simulink model "ES210A_EcuTMeas"  (R2013b)
settings: Solver=FixedStepDiscrete  SolverMode=SingleTasking  StartTime=0.0  StopTime=1  FixedStep=0.002  RelTol=1e-3
undefined symbols (not defined in the file): ARCHGLBPRM_100MILLISEC_SEC_F32, EcuTFild, EcuTMeasDftT, EcuTMeasFilTau, EcuTMeasNtc0x045FailStep, EcuTMeasNtc0x045PassStep, EcuTMeasRngDiagcMax, EcuTMeasRngDiagcMin, EcuTMeasScag, EcuTMeasScagOffs, NtcSts1, sigbuilder_block
libraries: simulink x2
settings Model: Creator=pz79n7  LastModifiedBy=NZG49T
settings SolverCC: AutoInsertRateTranBlk=on  InsertRTBMode=Always
settings DataIOCC: LimitDataPoints=off  SaveFormat=Structure  ReturnWorkspaceOutputs=on
settings OptimizationCC: BlockReduction=off  InlineParams=on  ZeroExternalMemoryAtStartup=off  ZeroInternalMemoryAtStartup=off  OptimizeModelRefInitCode=on  LifeSpan=1
settings DebuggingCC: SignalInfNanChecking=error  SignalRangeChecking=warning  UnderspecifiedInitializationDetection=Simplified  SolverPrmCheckMsg=error  InheritedTsInSrcMsg=error  DiscreteInheritContinuousMsg=error  SingleTaskRateTransMsg=error  TasksWithSamePriorityMsg=error  SigSpecEnsureSampleTimeMsg=error  CheckMatrixSingularityMsg=error  ParameterUnderflowMsg=error  ParameterPrecisionLossMsg=error  ParameterTunabilityLossMsg=error  FixptConstUnderflowMsg=warning  FixptConstOverflowMsg=warning  VectorMatrixConversionMsg=error  SignalLabelMismatchMsg=error  UnconnectedInputMsg=error  UnconnectedOutputMsg=error  UnconnectedLineMsg=error  SFcnCompatibilityMsg=error  UniqueDataStoreMsg=warning  BusObjectLabelMismatch=error  RootOutportRequireBusObject=error  AssertControl=DisableAll  ModelReferenceIOMsg=error  ModelReferenceVersionMismatchMessage=warning  ModelReferenceIOMismatchMessage=error  ModelReferenceCSMismatchMessage=warning  ModelReferenceDataLoggingMessage=error  StateNameClashWarn=warning  StrictBusMsg=ErrorOnBusTreatedAsVector  NonBusSignalsTreatedAsBus=error  SFUnexpectedBacktrackingDiag=error  SFInvalidInputDataAccessInChartInitDiag=error  SFNoUnconditionalDefaultTransitionDiag=error  SFTransitionOutsideNaturalParentDiag=error  SFUnconditionalTransitionShadowingDiag=error  SFUndirectedBroadcastEventsDiag=error
settings ModelReferenceCC: ModelReferenceNumInstancesAllowed=Single
settings RTWCC: SystemTargetFile=autosar.tlc  GenCodeOnly=on  TemplateMakefile=ert_default_tmf  Description=AUTOSAR  GenerateReport=on  ProcessScript=autosar_make_rtw_hook  LaunchReport=on
settings CodeAppCC: GenerateComments=off  IgnoreCustomStorageClasses=off  CustomSymbolStrType=$N$R$M  CustomSymbolStrBlkIO=$N$M  SimulinkBlockComments=off
settings STFCustomTargetCC: ParMdlRefBuildCompliant=on  CompOptLevelCompliant=on  IncludeMdlTerminateFcn=off  CombineOutputUpdateFcns=on  SuppressErrorStatus=on  ERTFirstTimeCompliant=on  ERTCustomFileBanners=on  SupportNonFinite=off  SupportComplex=off  SupportContinuousTime=off  SupportNonInlinedSFcns=off  MATLABClassNameForMDSCustomization=Simulink.SoftwareTarget.ERTCustomization  AutosarCompliant=on  GRTInterface=off  SystemTargetFile=autosar.tlc
settings ERTTargetCC: CodeReplacementLibrary=ANSI_C  ConcurrentExecutionCompliant=off  IncludeMdlTerminateFcn=off  SuppressErrorStatus=on  SupportNonFinite=off  SupportComplex=off  ModelStepFunctionPrototypeControlCompliant=off  CPPClassGenCompliant=off  AutosarCompliant=on  InlinedParameterPlacement=NonHierarchical  ERTCustomFileTemplate=example_file_process.tlc  EnableUserReplacementTypes=on

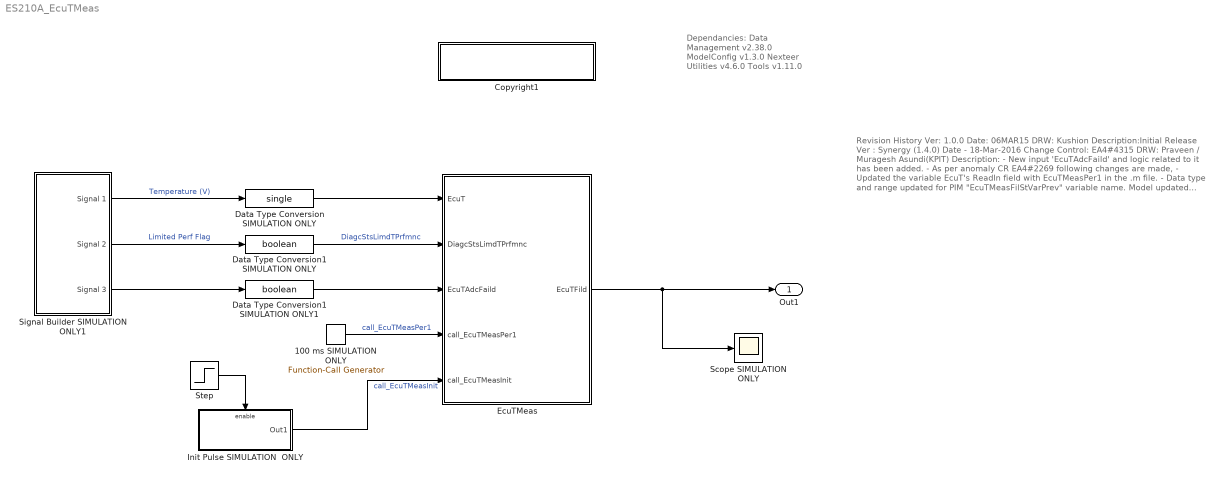
== system ES210A_EcuTMeas ==
  note: Dependancies:
      |    Data Management v2.38.0
      |    ModelConfig v1.3.0
      |    Nexteer Utilities v4.6.0
      |    Tools v1.11.0
  note: Revision History
      |
      | Ver: 1.0.0
      | Date: 06MAR15
      | DRW: Kushion
      | Description:Initial Release
      |
      | Ver : Synergy (1.4.0)
      | Date - 18-Mar-2016
      | Change Control: EA4#4315
      | DRW: Praveen / Muragesh Asundi(KPIT)
      | Description:
      | - New input 'EcuTAdcFaild' and logic related to it has been added.
      | -  As per anomaly CR EA4#2269 following changes are made,
      |   - Updated the variable EcuT's ReadIn field with EcuTMeasPer1 in the .m file.
      |   - Data type and range updated for PIM "EcuTMeasFilStVarPrev" variable name.
      |     Model updated accordingly
      |  - Global constant ARCHGLBPRM_100MILLISEC_SEC_F32 added
      |  - Requirements links updated
      |
      | Ver : 1.4.1
      | Date - 24-Mar-2016
      | Change Control: EA4#4947
      | DRW: Muragesh Asundi(KPIT)
      | New input 'EcuTAdcFaild' added in Data Dict
      |
      | Ver : 1.5.0
      | Date - 28-Apr-2016
      | Change Control: EA4#5549
      | DRW: Samanth Kumaraswamy
      | Changed the incorrect NTC number to 0x45
      | Changed .m file to reflect changes mentioned in the anomaly
      | Added new SetNtcSts Block for DebType for MIL Coverage
  100 ms SIMULATION ONLY : simulink/Ports & Subsystems/Function-Call Generator  sample_time=0.1  numberOfIterations=1
  Copyright1 : Subsystem  Description=|  mask(Copyright Information){none=on}
      | Copyright info block.                                               
      |                                                                     
      | Place copyright information at the top of every subsystem in design.
      mask prompts: none "No parameters"
      mask help: Place copyright information at the top of every subsystem in design.
      mask Display:
      | NxtrConf = 'Nexteer Confidential';
      | 
      | sys = bdroot; %handle for the current model ("system")
      | first = get_param(sys,'Created');
      | if(isempty(first))
      |     first = datestr(now,'yyyy');
      | else
      |     first = first(end-3:end);  %year is last four digits
      | end
      | 
      | last = get_param(sys,'LastModifiedDate');
      | if isempty(last)
      |     last = datestr(now,'yyyy');
      | else
      |     last = last(end-3:end);
      | end
      | 
      | if strcmp(first,last)
      |     fprintf('%s\nCopyright  %s Nexteer',NxtrConf,first);
      | else
      |     fprintf('%s\n%s%s-%s Nexteer',NxtrConf,char(169),first,last);
      | end
  Data Type Conversion SIMULATION ONLY : DataTypeConversion  OutDataTypeStr=single
  Data Type Conversion1 SIMULATION ONLY : DataTypeConversion  OutDataTypeStr=boolean
  Data Type Conversion1 SIMULATION ONLY1 : DataTypeConversion  OutDataTypeStr=boolean
  EcuTMeas : Subsystem
      settings: AttributesFormatString=ES210A
  Init Pulse SIMULATION  ONLY : Subsystem  TreatAsAtomicUnit=on
  Scope SIMULATION ONLY : Scope
      settings: YMin=-50  YMax=150
  Signal Builder SIMULATION ONLY1 : Subsystem  Tag=STV Subsys  LoadFcn=sigbuilder_block('load');  StartFcn=sigbuilder_block('start');  StopFcn=sigbuilder_block('stop');  ClipboardFcn=sigbuilder_block('clipboard');  mask(Sigbuilder block){}
      mask help: Simulink:masks:SigbuilderBlock_MD
      mask init:
      | if ~strcmp(get_param(bdroot(gcbh),'SimulationStatus'),'stopped') tuvar = sigbuilder_block('maskInit'); end
      settings: CopyFcn=sigbuilder_block('copy');  DeleteFcn=sigbuilder_block('delete');  ModelCloseFcn=sigbuilder_block('modelClose');  PreSaveFcn=sigbuilder_block('preSave');  PauseFcn=sigbuilder_block('pause');  ContinueFcn=sigbuilder_block('continue');  NameChangeFcn=sigbuilder_block('namechange');  OpenFcn=sigbuilder_block('open',[33 175.5 591 337.5 ]);  CloseFcn=sigbuilder_block('close');
      mask Display: plot(0, 0, 100, 100,[2, 2, 32, 32, 2], [68, 8, 8, 68, 68],[32, 2], [38, 38], [32, 19, 2],[53, 60, 44], [32, 17, 17, 2],[16, 16, 31, 31]);txt = getActiveGroup(gcbh);text(2, 100, txt,'verticalAlignment', 'top');
  Step : Step  Time=0.002  Before=1  After=0  SampleTime=0
  Out1 : Outport
  wires:
  Signal Builder SIMULATION ONLY1/1(Signal 1) -> Data Type Conversion SIMULATION ONLY/1  "Temperature (V)"
  Signal Builder SIMULATION ONLY1/2(Signal 2) -> Data Type Conversion1 SIMULATION ONLY/1  "Limited Perf Flag"
  100 ms SIMULATION ONLY/1 -> EcuTMeas/4(call_EcuTMeasPer1)  "call_EcuTMeasPer1"
  Step/1 -> Init Pulse SIMULATION  ONLY/Enable
  Init Pulse SIMULATION  ONLY/1(Out1) -> EcuTMeas/5(call_EcuTMeasInit)  "call_EcuTMeasInit"
  Data Type Conversion SIMULATION ONLY/1 -> EcuTMeas/1(EcuT)
  Data Type Conversion1 SIMULATION ONLY/1 -> EcuTMeas/2(DiagcStsLimdTPrfmnc)  "DiagcStsLimdTPrfmnc"
  EcuTMeas/1(EcuTFild) -> Scope SIMULATION ONLY/1, Out1/1
  Signal Builder SIMULATION ONLY1/3(Signal 3) -> Data Type Conversion1 SIMULATION ONLY1/1
  Data Type Conversion1 SIMULATION ONLY1/1 -> EcuTMeas/3(EcuTAdcFaild)

== system ES210A_EcuTMeas/Copyright1 ==

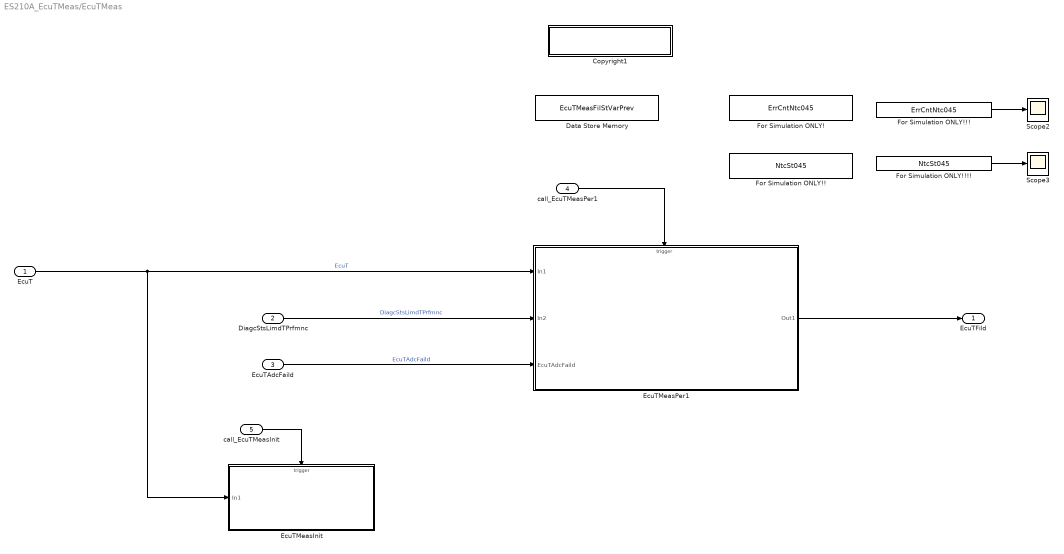
== system ES210A_EcuTMeas/EcuTMeas ==
  EcuT : Inport  RequirementInfo={'linktype_rmi_doors' '000089bf (/E-STEER Core/SubSystem Specifications/Electrical Actuator/Control Module/FDD Module Requirements/EA4/ES210A_EcuTMeas)' '#ES210A_48' 'true' 'REQ: ES210A_48' '' } %GIDa_562c6c3c_e149_4b8a_bc2f_eb7571733cee
  DiagcStsLimdTPrfmnc : Inport  RequirementInfo={'linktype_rmi_doors' '000089bf (/E-STEER Core/SubSystem Specifications/Electrical Actuator/Control Module/FDD Module Requirements/EA4/ES210A_EcuTMeas)' '#ES210A_71' 'true' 'REQ: ES210A_71' '' } %GIDa_c32b2e62_ca29_48d9_a45f_43e18439e176  Port=2
  EcuTAdcFaild : Inport  RequirementInfo={'linktype_rmi_doors' '000089bf (/E-STEER Core/SubSystem Specifications/Electrical Actuator/Control Module/FDD Module Requirements/EA4/ES210A_EcuTMeas)' '#ES210A_82' 'true' 'REQ: ES210A_82' '' } %GIDa_33c9adb4_3b4d_41a0_b691_c5854dca2733  Port=3
  call_EcuTMeasPer1 : Inport  RequirementInfo={'linktype_rmi_doors' '000089bf (/E-STEER Core/SubSystem Specifications/Electrical Actuator/Control Module/FDD Module Requirements/EA4/ES210A_EcuTMeas)' '#ES210A_81' 'true' 'REQ: ES210A_81' '' ; 'linktype_rmi_doors' '000089bf (/E-STEER Core/SubSystem Specifications/Electrical Actuator/Control Module/FDD Module Requirements/EA4/ES210A_EcuTMeas)' '#ES210A_25' 'true' 'REQ: ES210A_25' '' } %GIDa_ca696ddf_736a_4d4a_b70f_f10e14ff3279  Port=4
  call_EcuTMeasInit : Inport  Port=5
  Copyright1 : Subsystem  Description=|  mask(Copyright Information){none=on}
      | Copyright info block.                                               
      |                                                                     
      | Place copyright information at the top of every subsystem in design.
      mask prompts: none "No parameters"
      mask help: Place copyright information at the top of every subsystem in design.
      mask Display:
      | NxtrConf = 'Nexteer Confidential';
      | 
      | sys = bdroot; %handle for the current model ("system")
      | first = get_param(sys,'Created');
      | if(isempty(first))
      |     first = datestr(now,'yyyy');
      | else
      |     first = first(end-3:end);  %year is last four digits
      | end
      | 
      | last = get_param(sys,'LastModifiedDate');
      | if isempty(last)
      |     last = datestr(now,'yyyy');
      | else
      |     last = last(end-3:end);
      | end
      | 
      | if strcmp(first,last)
      |     fprintf('%s\nCopyright  %s Nexteer',NxtrConf,first);
      | else
      |     fprintf('%s\n%s%s-%s Nexteer',NxtrConf,char(169),first,last);
      | end
  Data Store Memory : DataStoreMemory  DataStoreName=EcuTMeasFilStVarPrev  InitialValue=struct('FilSt',single(0),'FilGain',single(0))  OutDataTypeStr=Bus: FilLpRec1  StateMustResolveToSignalObject=on
  EcuTMeasInit : Subsystem  RequirementInfo={'linktype_rmi_doors' '000089bf (/E-STEER Core/SubSystem Specifications/Electrical Actuator/Control Module/FDD Module Requirements/EA4/ES210A_EcuTMeas)' '#ES210A_80' 'true' 'REQ: ES210A_80' '' } %GIDa_ede09633_558d_45b8_b146_d426592bfdd4  TreatAsAtomicUnit=on
  EcuTMeasPer1 : Subsystem  TreatAsAtomicUnit=on
  For Simulation ONLY! : DataStoreMemory  DataStoreName=ErrCntNtc045
  For Simulation ONLY!! : DataStoreMemory  DataStoreName=NtcSt045  OutDataTypeStr=uint8
  For Simulation ONLY!!! : DataStoreRead  DataStoreName=ErrCntNtc045  SampleTime=0.1
  For Simulation ONLY!!!! : DataStoreRead  DataStoreName=NtcSt045  SampleTime=0.1
  Scope2 : Scope
      settings: YMin=-35000  YMax=35000  SaveName=ScopeData2  MaxDataPoints=20000
  Scope3 : Scope
      settings: YMin=-35000  YMax=5000  SaveName=ScopeData4  MaxDataPoints=20000
  EcuTFild : Outport  RequirementInfo={'linktype_rmi_doors' '000089bf (/E-STEER Core/SubSystem Specifications/Electrical Actuator/Control Module/FDD Module Requirements/EA4/ES210A_EcuTMeas)' '#ES210A_51' 'true' 'REQ: ES210A_51' '' } %GIDa_e5beccf4_d72f_4678_b409_538621bbf562
  wires:
  EcuT/1 -> EcuTMeasInit/1(In1), EcuTMeasPer1/1(In1)  "EcuT"
  DiagcStsLimdTPrfmnc/1 -> EcuTMeasPer1/2(In2)  "DiagcStsLimdTPrfmnc"
  EcuTMeasPer1/1(Out1) -> EcuTFild/1
  call_EcuTMeasPer1/1 -> EcuTMeasPer1/Trigger
  call_EcuTMeasInit/1 -> EcuTMeasInit/Trigger
  For Simulation ONLY!!!/1 -> Scope2/1
  For Simulation ONLY!!!!/1 -> Scope3/1
  EcuTAdcFaild/1 -> EcuTMeasPer1/3(EcuTAdcFaild)  "EcuTAdcFaild"

== system ES210A_EcuTMeas/Init Pulse SIMULATION  ONLY ==
  Enable : EnablePort
  "0.002 " : simulink/Ports & Subsystems/Function-Call Generator  sample_time=0.002  numberOfIterations=1
  Copyright1 : Subsystem  Description=|  mask(Copyright Information){none=on}
      | Copyright info block.                                               
      |                                                                     
      | Place copyright information at the top of every subsystem in design.
      mask prompts: none "No parameters"
      mask help: Place copyright information at the top of every subsystem in design.
      mask Display:
      | NxtrConf = 'Nexteer Confidential';
      | 
      | sys = bdroot; %handle for the current model ("system")
      | first = get_param(sys,'Created');
      | if(isempty(first))
      |     first = datestr(now,'yyyy');
      | else
      |     first = first(end-3:end);  %year is last four digits
      | end
      | 
      | last = get_param(sys,'LastModifiedDate');
      | if isempty(last)
      |     last = datestr(now,'yyyy');
      | else
      |     last = last(end-3:end);
      | end
      | 
      | if strcmp(first,last)
      |     fprintf('%s\nCopyright  %s Nexteer',NxtrConf,first);
      | else
      |     fprintf('%s\n%s%s-%s Nexteer',NxtrConf,char(169),first,last);
      | end
  Out1 : Outport
  wires:
  "0.002 "/1 -> Out1/1

== system ES210A_EcuTMeas/Signal Builder SIMULATION ONLY1 ==
  Demux : Demux  Tag=STV Demux  Outputs=3
  FromWs : FromWorkspace  Tag=STV FromWs  VariableName=tuvar  SampleTime=0
      SigBuilderData=|
      | common.afterFinalStr = 'Extrapolate'
      | common.sampleTime = 0
      | dataSet.timeRange = [0 20]
      | dataSet.name = 'Group 1'
      | sbobj.Groups.Name = 'Group 1'
      | sbobj.Groups.Signals(1).Name = 'Signal 1'
      | sbobj.Groups.Signals(1).XData = [0 0.44 0.44 4.05 6 10 20]
      | sbobj.Groups.Signals(1).YData = [0.1 0.1 2 1.98 0 -0.02 0.98]
      | sbobj.Groups.Signals(2).Name = 'Signal 2'
      | sbobj.Groups.Signals(2).XData = [0 12 12 16 16 20]
      | sbobj.Groups.Signals(2).YData = [0 0 1 1 0 0]
      | sbobj.Groups.Signals(3).Name = 'Signal 3'
      | sbobj.Groups.Signals(3).XData = [0 10 10 20]
      | sbobj.Groups.Signals(3).YData = [0 0 1 1]
      | sbobj.Groups.TimeRange = [0 20]
  Signal 1 : Outport  Tag=STV Outport
  Signal 2 : Outport  Tag=STV Outport  Port=2
  Signal 3 : Outport  Tag=STV Outport  Port=3
  wires:
  Demux/1 -> Signal 1/1
  FromWs/1 -> Demux/1
  Demux/2 -> Signal 2/1
  Demux/3 -> Signal 3/1

== system ES210A_EcuTMeas/EcuTMeas/Copyright1 ==

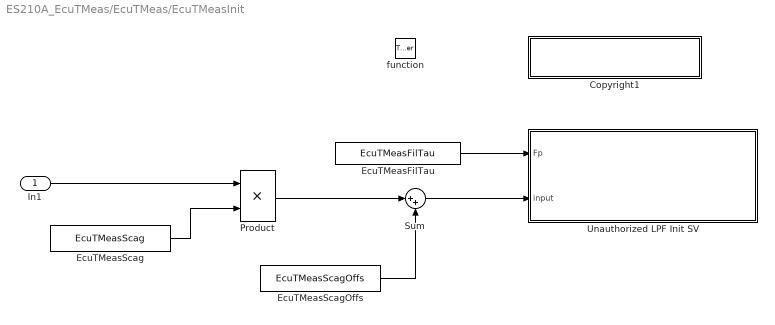
== system ES210A_EcuTMeas/EcuTMeas/EcuTMeasInit ==
  In1 : Inport
  function : TriggerPort  TriggerType=function-call
  Copyright1 : Subsystem  Description=|  mask(Copyright Information){none=on}
      | Copyright info block.                                               
      |                                                                     
      | Place copyright information at the top of every subsystem in design.
      mask prompts: none "No parameters"
      mask help: Place copyright information at the top of every subsystem in design.
      mask Display:
      | NxtrConf = 'Nexteer Confidential';
      | 
      | sys = bdroot; %handle for the current model ("system")
      | first = get_param(sys,'Created');
      | if(isempty(first))
      |     first = datestr(now,'yyyy');
      | else
      |     first = first(end-3:end);  %year is last four digits
      | end
      | 
      | last = get_param(sys,'LastModifiedDate');
      | if isempty(last)
      |     last = datestr(now,'yyyy');
      | else
      |     last = last(end-3:end);
      | end
      | 
      | if strcmp(first,last)
      |     fprintf('%s\nCopyright  %s Nexteer',NxtrConf,first);
      | else
      |     fprintf('%s\n%s%s-%s Nexteer',NxtrConf,char(169),first,last);
      | end
  EcuTMeasFilTau : Constant  RequirementInfo={'linktype_rmi_doors' '000089bf (/E-STEER Core/SubSystem Specifications/Electrical Actuator/Control Module/FDD Module Requirements/EA4/ES210A_EcuTMeas)' '#ES210A_67' 'true' 'REQ: ES210A_67' '' } %GIDa_f1dce8fb_aef4_4cc7_a37f_61aa5bf3e739  Value=EcuTMeasFilTau
  EcuTMeasScag : Constant  RequirementInfo={} %GIDa_ff96598e_3599_4953_8511_9f6c43a5e0a1  Value=EcuTMeasScag
  EcuTMeasScagOffs : Constant  RequirementInfo={} %GIDa_8b7473a9_4ab2_46d8_9d94_f7d56c34d4f4  Value=EcuTMeasScagOffs
  Product : Product  RequirementInfo={} %GIDa_a162ff9c_cdae_4af1_a9a0_ea0d92bfda14
  Sum : Sum  RequirementInfo={} %GIDa_ba1681a0_b4a7_47a3_b5b1_4ffa2c281a80  Inputs=|++
  Unauthorized LPF Init SV : Subsystem
  wires:
  EcuTMeasFilTau/1 -> Unauthorized LPF Init SV/1(Fp)
  In1/1 -> Product/1
  EcuTMeasScag/1 -> Product/2
  Product/1 -> Sum/1
  EcuTMeasScagOffs/1 -> Sum/2
  Sum/1 -> Unauthorized LPF Init SV/2(input)

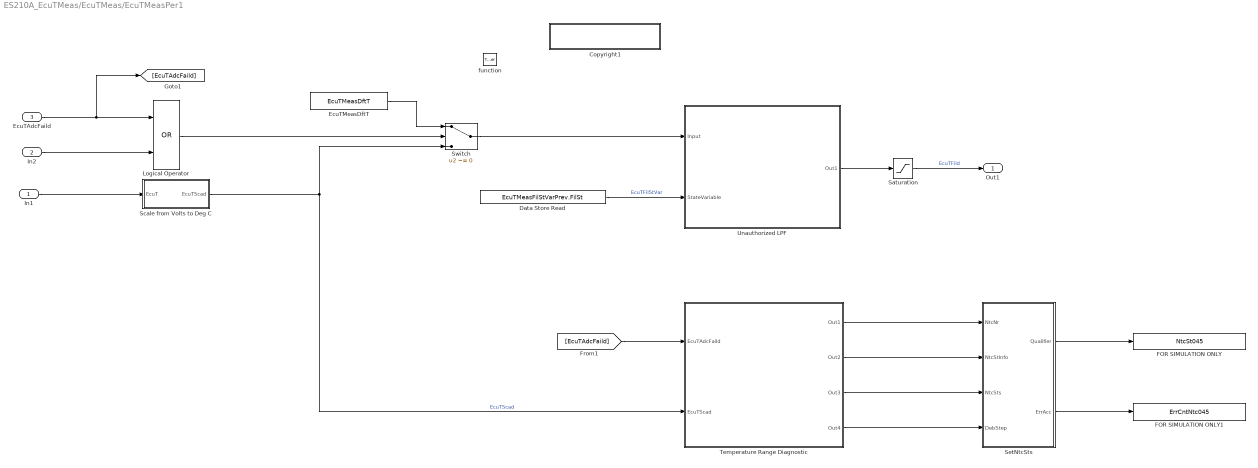
== system ES210A_EcuTMeas/EcuTMeas/EcuTMeasPer1 ==
  In1 : Inport
  In2 : Inport  Port=2
  EcuTAdcFaild : Inport  Port=3
  function : TriggerPort  TriggerType=function-call
  Copyright1 : Subsystem  Description=|  mask(Copyright Information){none=on}
      | Copyright info block.                                               
      |                                                                     
      | Place copyright information at the top of every subsystem in design.
      mask prompts: none "No parameters"
      mask help: Place copyright information at the top of every subsystem in design.
      mask Display:
      | NxtrConf = 'Nexteer Confidential';
      | 
      | sys = bdroot; %handle for the current model ("system")
      | first = get_param(sys,'Created');
      | if(isempty(first))
      |     first = datestr(now,'yyyy');
      | else
      |     first = first(end-3:end);  %year is last four digits
      | end
      | 
      | last = get_param(sys,'LastModifiedDate');
      | if isempty(last)
      |     last = datestr(now,'yyyy');
      | else
      |     last = last(end-3:end);
      | end
      | 
      | if strcmp(first,last)
      |     fprintf('%s\nCopyright  %s Nexteer',NxtrConf,first);
      | else
      |     fprintf('%s\n%s%s-%s Nexteer',NxtrConf,char(169),first,last);
      | end
  Data Store Read : DataStoreRead  DataStoreName=EcuTMeasFilStVarPrev  DataStoreElements=EcuTMeasFilStVarPrev.FilSt
  EcuTMeasDftT : Constant  RequirementInfo={'linktype_rmi_doors' '000089bf (/E-STEER Core/SubSystem Specifications/Electrical Actuator/Control Module/FDD Module Requirements/EA4/ES210A_EcuTMeas)' '#ES210A_84' 'true' 'REQ: ES210A_84' '' } %GIDa_b1347350_8d2d_43af_8bf2_ecc8e1b64997  Value=EcuTMeasDftT
  FOR SIMULATION ONLY : DataStoreWrite  DataStoreName=NtcSt045
  FOR SIMULATION ONLY1 : DataStoreWrite  DataStoreName=ErrCntNtc045
  Logical Operator : Logic  RequirementInfo={'linktype_rmi_doors' '000089bf (/E-STEER Core/SubSystem Specifications/Electrical Actuator/Control Module/FDD Module Requirements/EA4/ES210A_EcuTMeas)' '#ES210A_84' 'true' 'REQ: ES210A_84' '' } %GIDa_55355c33_b558_4344_8719_63703848629b  Operator=OR  AllPortsSameDT=off  OutDataTypeStr=boolean
  Saturation : Saturate  RequirementInfo={'linktype_rmi_doors' '000089bf (/E-STEER Core/SubSystem Specifications/Electrical Actuator/Control Module/FDD Module Requirements/EA4/ES210A_EcuTMeas)' '#ES210A_69' 'true' 'REQ: ES210A_69' '' } %GIDa_bc286417_5809_4236_bb31_07a4e8e6097f  UpperLimit=EcuTFild.EngMax  LowerLimit=EcuTFild.EngMin
  Scale from Volts to Deg C : Subsystem  RequirementInfo={'linktype_rmi_doors' '000089bf (/E-STEER Core/SubSystem Specifications/Electrical Actuator/Control Module/FDD Module Requirements/EA4/ES210A_EcuTMeas)' '#ES210A_68' 'true' 'REQ: ES210A_68' '' } %GIDa_c46bfcd3_545a_4c79_9c94_fb0d46bf8024
  SetNtcSts : Subsystem  RequirementInfo={} %GIDa_356baa60_f045_46f7_87ae_17993bf66008
      settings: RTWSystemCode=Inline
  Switch : Switch  Criteria=u2 ~= 0  Threshold=0.5
  Temperature Range Diagnostic : Subsystem  RequirementInfo={'linktype_rmi_doors' '000089bf (/E-STEER Core/SubSystem Specifications/Electrical Actuator/Control Module/FDD Module Requirements/EA4/ES210A_EcuTMeas)' '#ES210A_25' 'true' 'REQ: ES210A_25' '' } %GIDa_17485928_1225_48ba_bef0_e7c15712ebfb
  Unauthorized LPF : Subsystem  RequirementInfo={'linktype_rmi_doors' '000089bf (/E-STEER Core/SubSystem Specifications/Electrical Actuator/Control Module/FDD Module Requirements/EA4/ES210A_EcuTMeas)' '#ES210A_67' 'true' 'REQ: ES210A_67' '' } %GIDa_c4c8dad2_b6d2_48c5_a43c_d6758f2cdb0e
  Out1 : Outport
  wires:
  Scale from Volts to Deg C/1(EcuTScad) -> Temperature Range Diagnostic/2(EcuTScad), Switch/3  "EcuTScad"
  In2/1 -> Logical Operator/2
  EcuTMeasDftT/1 -> Switch/1
  Switch/1 -> Unauthorized LPF/1(Input)
  Unauthorized LPF/1(Out1) -> Saturation/1
  Saturation/1 -> Out1/1  "EcuTFild"
  Data Store Read/1 -> Unauthorized LPF/2(StateVariable)  "EcuTFilStVar"
  Temperature Range Diagnostic/1(Out1) -> SetNtcSts/1(NtcNr)
  Temperature Range Diagnostic/2(Out2) -> SetNtcSts/2(NtcStInfo)
  Temperature Range Diagnostic/3(Out3) -> SetNtcSts/3(NtcSts)
  Temperature Range Diagnostic/4(Out4) -> SetNtcSts/4(DebStep)
  SetNtcSts/1(Qualifier) -> FOR SIMULATION ONLY/1
  SetNtcSts/2(ErrAcc) -> FOR SIMULATION ONLY1/1
  In1/1 -> Scale from Volts to Deg C/1(EcuT)
  EcuTAdcFaild/1 -> [EcuTAdcFaild], Logical Operator/1
  Logical Operator/1 -> Switch/2
  [EcuTAdcFaild] -> Temperature Range Diagnostic/1(EcuTAdcFaild)

== system ES210A_EcuTMeas/Init Pulse SIMULATION  ONLY/Copyright1 ==

== system ES210A_EcuTMeas/EcuTMeas/EcuTMeasInit/Copyright1 ==

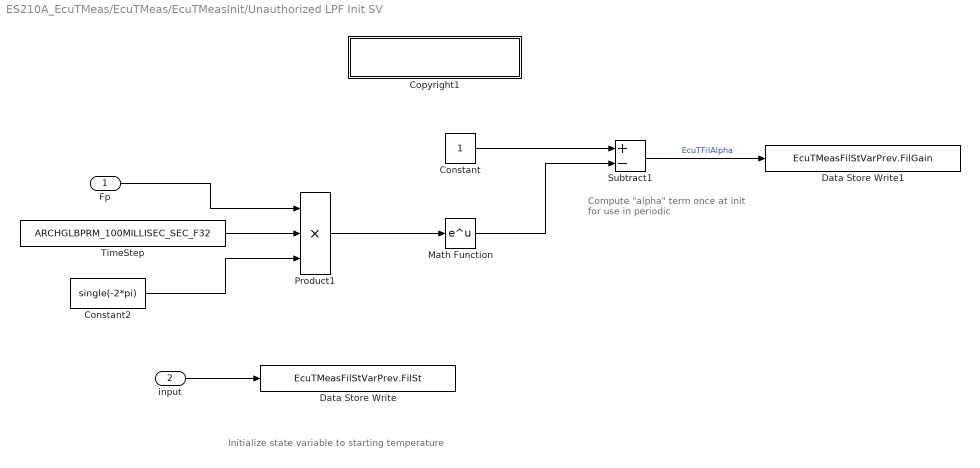
== system ES210A_EcuTMeas/EcuTMeas/EcuTMeasInit/Unauthorized LPF Init SV ==
  note: Compute "alpha" term once at init
      | for use in periodic
  note: Initialize state variable to starting temperature
  Fp : Inport  OutDataTypeStr=single
  input : Inport  Port=2  OutDataTypeStr=single
  Constant : Constant  OutDataTypeStr=single
  Constant2 : Constant  Value=single(-2*pi)  OutDataTypeStr=single
  Copyright1 : Subsystem  Description=|  mask(Copyright Information){none=on}
      | Copyright info block.                                               
      |                                                                     
      | Place copyright information at the top of every subsystem in design.
      mask prompts: none "No parameters"
      mask help: Place copyright information at the top of every subsystem in design.
      mask Display:
      | NxtrConf = 'Nexteer Confidential';
      | 
      | sys = bdroot; %handle for the current model ("system")
      | first = get_param(sys,'Created');
      | if(isempty(first))
      |     first = datestr(now,'yyyy');
      | else
      |     first = first(end-3:end);  %year is last four digits
      | end
      | 
      | last = get_param(sys,'LastModifiedDate');
      | if isempty(last)
      |     last = datestr(now,'yyyy');
      | else
      |     last = last(end-3:end);
      | end
      | 
      | if strcmp(first,last)
      |     fprintf('%s\nCopyright  %s Nexteer',NxtrConf,first);
      | else
      |     fprintf('%s\n%s%s-%s Nexteer',NxtrConf,char(169),first,last);
      | end
  Data Store Write : DataStoreWrite  DataStoreName=EcuTMeasFilStVarPrev  DataStoreElements=EcuTMeasFilStVarPrev.FilSt
  Data Store Write1 : DataStoreWrite  DataStoreName=EcuTMeasFilStVarPrev  DataStoreElements=EcuTMeasFilStVarPrev.FilGain
  Math Function : Math  SaturateOnIntegerOverflow=on
  Product1 : Product  Inputs=3
  Subtract1 : Sum  Inputs=+-
  TimeStep : Constant  Value=ARCHGLBPRM_100MILLISEC_SEC_F32  OutDataTypeStr=single
  wires:
  Constant2/1 -> Product1/3
  Product1/1 -> Math Function/1
  TimeStep/1 -> Product1/2
  Math Function/1 -> Subtract1/2
  Constant/1 -> Subtract1/1
  input/1 -> Data Store Write/1
  Subtract1/1 -> Data Store Write1/1  "EcuTFilAlpha"
  Fp/1 -> Product1/1

== system ES210A_EcuTMeas/EcuTMeas/EcuTMeasPer1/Copyright1 ==

== system ES210A_EcuTMeas/EcuTMeas/EcuTMeasPer1/Scale from Volts to Deg C ==
  EcuT : Inport
  EcuTMeasScag : Constant  RequirementInfo={} %GIDa_fcba7590_e467_4009_a0d3_e989568603e9  Value=EcuTMeasScag
  EcuTMeasScagOffs : Constant  RequirementInfo={} %GIDa_b5444b8f_5f71_4a0d_9313_d7843e97597d  Value=EcuTMeasScagOffs
  Product : Product  RequirementInfo={} %GIDa_258f3aed_d36f_4cfe_8be3_25a8bd5f7d9a
  Sum : Sum  RequirementInfo={} %GIDa_6fe0701f_435c_4bf6_94a1_324a38b136d9  Inputs=|++
  EcuTScad : Outport
  wires:
  EcuT/1 -> Product/1
  EcuTMeasScag/1 -> Product/2
  Product/1 -> Sum/1
  EcuTMeasScagOffs/1 -> Sum/2
  Sum/1 -> EcuTScad/1  "EcuTScad"

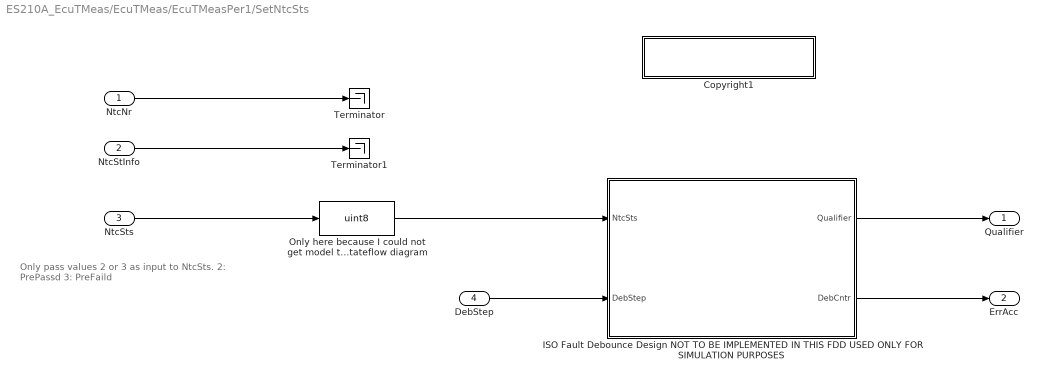
== system ES210A_EcuTMeas/EcuTMeas/EcuTMeasPer1/SetNtcSts ==
  note: Only pass values 2 or 3 as input to NtcSts.
      | 2: PrePassd
      | 3: PreFaild
  NtcNr : Inport
  NtcStInfo : Inport  Port=2
  NtcSts : Inport  Port=3
  DebStep : Inport  Port=4
  Copyright1 : Subsystem  Description=|  mask(Copyright Information){none=on}
      | Copyright info block.                                               
      |                                                                     
      | Place copyright information at the top of every subsystem in design.
      mask prompts: none "No parameters"
      mask help: Place copyright information at the top of every subsystem in design.
      mask Display:
      | NxtrConf = 'Nexteer Confidential';
      | 
      | sys = bdroot; %handle for the current model ("system")
      | first = get_param(sys,'Created');
      | if(isempty(first))
      |     first = datestr(now,'yyyy');
      | else
      |     first = first(end-3:end);  %year is last four digits
      | end
      | 
      | last = get_param(sys,'LastModifiedDate');
      | if isempty(last)
      |     last = datestr(now,'yyyy');
      | else
      |     last = last(end-3:end);
      | end
      | 
      | if strcmp(first,last)
      |     fprintf('%s\nCopyright  %s Nexteer',NxtrConf,first);
      | else
      |     fprintf('%s\n%s%s-%s Nexteer',NxtrConf,char(169),first,last);
      | end
  ISO Fault Debounce Design NOT TO BE IMPLEMENTED IN THIS FDD USED ONLY FOR SIMULATION PURPOSES : Stateflow chart  TreatAsAtomicUnit=on
  Only here because I could not get model to run with enumerations in the stateflow diagram : DataTypeConversion  OutDataTypeStr=uint8
  Terminator : Terminator
  Terminator1 : Terminator
  Qualifier : Outport
  ErrAcc : Outport  Port=2
  wires:
  NtcStInfo/1 -> Terminator1/1
  NtcNr/1 -> Terminator/1
  NtcSts/1 -> Only here because I could not get model to run with enumerations in the stateflow diagram/1
  DebStep/1 -> ISO Fault Debounce Design NOT TO BE IMPLEMENTED IN THIS FDD USED ONLY FOR SIMULATION PURPOSES/2(DebStep)
  ISO Fault Debounce Design NOT TO BE IMPLEMENTED IN THIS FDD USED ONLY FOR SIMULATION PURPOSES/1(Qualifier) -> Qualifier/1
  Only here because I could not get model to run with enumerations in the stateflow diagram/1 -> ISO Fault Debounce Design NOT TO BE IMPLEMENTED IN THIS FDD USED ONLY FOR SIMULATION PURPOSES/1(NtcSts)
  ISO Fault Debounce Design NOT TO BE IMPLEMENTED IN THIS FDD USED ONLY FOR SIMULATION PURPOSES/2(DebCntr) -> ErrAcc/1

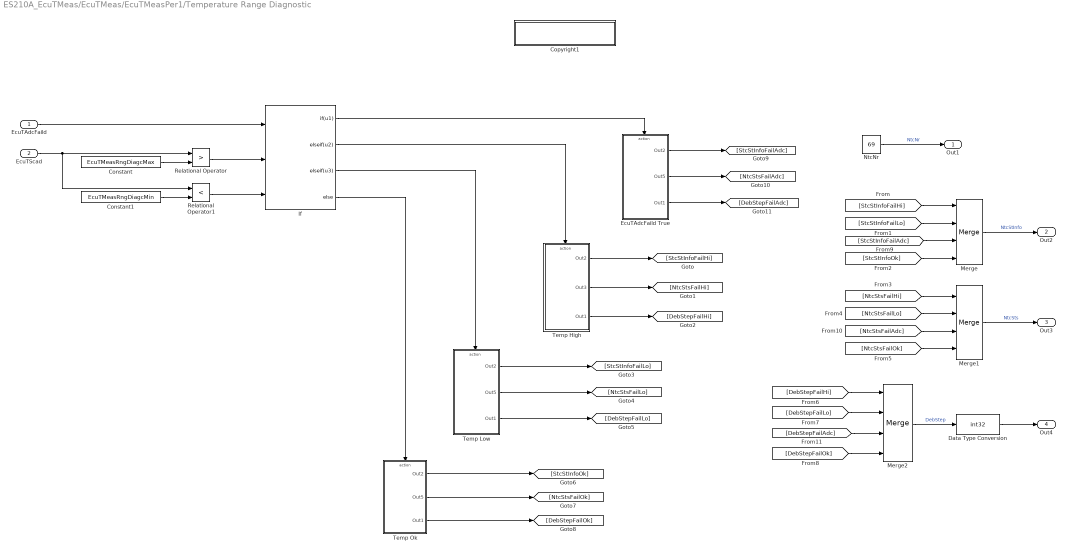
== system ES210A_EcuTMeas/EcuTMeas/EcuTMeasPer1/Temperature Range Diagnostic ==
  EcuTAdcFaild : Inport
  EcuTScad : Inport  Port=2
  Constant : Constant  Value=EcuTMeasRngDiagcMax
  Constant1 : Constant  Value=EcuTMeasRngDiagcMin
  Copyright1 : Subsystem  Description=|  mask(Copyright Information){none=on}
      | Copyright info block.                                               
      |                                                                     
      | Place copyright information at the top of every subsystem in design.
      mask prompts: none "No parameters"
      mask help: Place copyright information at the top of every subsystem in design.
      mask Display:
      | NxtrConf = 'Nexteer Confidential';
      | 
      | sys = bdroot; %handle for the current model ("system")
      | first = get_param(sys,'Created');
      | if(isempty(first))
      |     first = datestr(now,'yyyy');
      | else
      |     first = first(end-3:end);  %year is last four digits
      | end
      | 
      | last = get_param(sys,'LastModifiedDate');
      | if isempty(last)
      |     last = datestr(now,'yyyy');
      | else
      |     last = last(end-3:end);
      | end
      | 
      | if strcmp(first,last)
      |     fprintf('%s\nCopyright  %s Nexteer',NxtrConf,first);
      | else
      |     fprintf('%s\n%s%s-%s Nexteer',NxtrConf,char(169),first,last);
      | end
  Data Type Conversion : DataTypeConversion  OutDataTypeStr=int32
  EcuTAdcFaild True : Subsystem  RequirementInfo={'linktype_rmi_doors' '000089bf (/E-STEER Core/SubSystem Specifications/Electrical Actuator/Control Module/FDD Module Requirements/EA4/ES210A_EcuTMeas)' '#ES210A_83' 'true' 'REQ: ES210A_83' '' } %GIDa_e5d583f1_a319_4d28_b962_955d1e9a2005  TreatAsAtomicUnit=on
  If : If  NumInputs=3  IfExpression=u1  ElseIfExpressions=u2, u3
  Merge : Merge  Inputs=4
  Merge1 : Merge  Inputs=4
  Merge2 : Merge  Inputs=4
  NtcNr : Constant  Value=69
  Relational Operator : RelationalOperator  Operator=>  OutDataTypeStr=boolean
  Relational Operator1 : RelationalOperator  Operator=<  OutDataTypeStr=boolean
  Temp High : Subsystem  RequirementInfo={'linktype_rmi_doors' '000089bf (/E-STEER Core/SubSystem Specifications/Electrical Actuator/Control Module/FDD Module Requirements/EA4/ES210A_EcuTMeas)' '#ES210A_28' 'true' 'REQ: ES210A_28' '' ; 'linktype_rmi_doors' '000089bf (/E-STEER Core/SubSystem Specifications/Electrical Actuator/Control Module/FDD Module Requirements/EA4/ES210A_EcuTMeas)' '#ES210A_69' 'true' 'REQ: ES210A_69' '' } %GIDa_f4070c03_e9e6_43a9_a48d_e5a89d0a3f64  TreatAsAtomicUnit=on
  Temp Low : Subsystem  RequirementInfo={'linktype_rmi_doors' '000089bf (/E-STEER Core/SubSystem Specifications/Electrical Actuator/Control Module/FDD Module Requirements/EA4/ES210A_EcuTMeas)' '#ES210A_69' 'true' 'REQ: ES210A_69' '' ; 'linktype_rmi_doors' '000089bf (/E-STEER Core/SubSystem Specifications/Electrical Actuator/Control Module/FDD Module Requirements/EA4/ES210A_EcuTMeas)' '#ES210A_70' 'true' 'REQ: ES210A_70' '' } %GIDa_875aeff0_490d_436d_8737_d5dcd122b0c2  TreatAsAtomicUnit=on
  Temp Ok : Subsystem  RequirementInfo={'linktype_rmi_doors' '000089bf (/E-STEER Core/SubSystem Specifications/Electrical Actuator/Control Module/FDD Module Requirements/EA4/ES210A_EcuTMeas)' '#ES210A_31' 'true' 'REQ: ES210A_31' '' } %GIDa_6226e280_34ba_404c_a5f1_1f5eac1f837a  TreatAsAtomicUnit=on
  Out1 : Outport
  Out2 : Outport  Port=2
  Out3 : Outport  Port=3
  Out4 : Outport  Port=4
  wires:
  If/4 -> Temp Ok/Action
  NtcNr/1 -> Out1/1  "NtcNr"
  Merge/1 -> Out2/1  "NtcStInfo"
  Temp High/1(Out2) -> [StcStInfoFailHi]
  Temp High/2(Out3) -> [NtcStsFailHi]
  Temp High/3(Out1) -> [DebStepFailHi]
  Temp Low/1(Out2) -> [StcStInfoFailLo]
  Temp Low/2(Out5) -> [NtcStsFailLo]
  Temp Low/3(Out1) -> [DebStepFailLo]
  Temp Ok/1(Out2) -> [StcStInfoOk]
  Temp Ok/2(Out5) -> [NtcStsFailOk]
  Temp Ok/3(Out1) -> [DebStepFailOk]
  [StcStInfoFailHi] -> Merge/1
  [StcStInfoFailLo] -> Merge/2
  Merge1/1 -> Out3/1  "NtcSts"
  [NtcStsFailHi] -> Merge1/1
  [NtcStsFailLo] -> Merge1/2
  Merge2/1 -> Data Type Conversion/1  "DebStep"
  [DebStepFailHi] -> Merge2/1
  [DebStepFailLo] -> Merge2/2
  Data Type Conversion/1 -> Out4/1
  EcuTAdcFaild/1 -> If/1
  EcuTScad/1 -> Relational Operator1/1, Relational Operator/1
  Relational Operator/1 -> If/2
  Constant/1 -> Relational Operator/2
  Constant1/1 -> Relational Operator1/2
  Relational Operator1/1 -> If/3
  If/3 -> Temp Low/Action
  If/2 -> Temp High/Action
  If/1 -> EcuTAdcFaild True/Action
  EcuTAdcFaild True/1(Out2) -> [StcStInfoFailAdc]
  EcuTAdcFaild True/2(Out5) -> [NtcStsFailAdc]
  EcuTAdcFaild True/3(Out1) -> [DebStepFailAdc]
  [StcStInfoFailAdc] -> Merge/3
  [StcStInfoOk] -> Merge/4
  [NtcStsFailAdc] -> Merge1/3
  [NtcStsFailOk] -> Merge1/4
  [DebStepFailOk] -> Merge2/4
  [DebStepFailAdc] -> Merge2/3

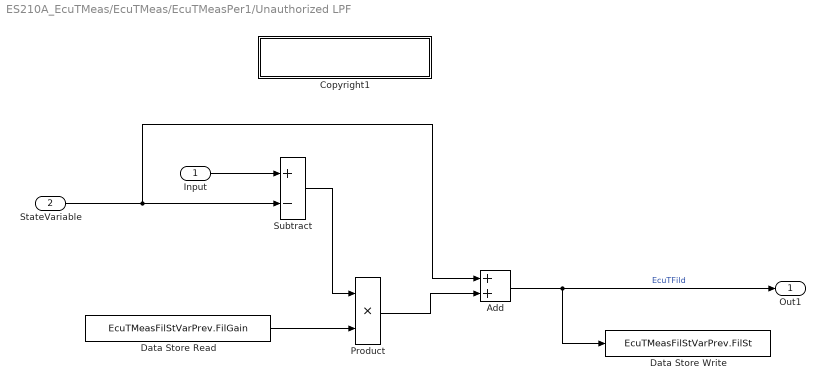
== system ES210A_EcuTMeas/EcuTMeas/EcuTMeasPer1/Unauthorized LPF ==
  Input : Inport
  StateVariable : Inport  Port=2
  Add : Sum
  Copyright1 : Subsystem  Description=|  mask(Copyright Information){none=on}
      | Copyright info block.                                               
      |                                                                     
      | Place copyright information at the top of every subsystem in design.
      mask prompts: none "No parameters"
      mask help: Place copyright information at the top of every subsystem in design.
      mask Display:
      | NxtrConf = 'Nexteer Confidential';
      | 
      | sys = bdroot; %handle for the current model ("system")
      | first = get_param(sys,'Created');
      | if(isempty(first))
      |     first = datestr(now,'yyyy');
      | else
      |     first = first(end-3:end);  %year is last four digits
      | end
      | 
      | last = get_param(sys,'LastModifiedDate');
      | if isempty(last)
      |     last = datestr(now,'yyyy');
      | else
      |     last = last(end-3:end);
      | end
      | 
      | if strcmp(first,last)
      |     fprintf('%s\nCopyright  %s Nexteer',NxtrConf,first);
      | else
      |     fprintf('%s\n%s%s-%s Nexteer',NxtrConf,char(169),first,last);
      | end
  Data Store Read : DataStoreRead  DataStoreName=EcuTMeasFilStVarPrev  DataStoreElements=EcuTMeasFilStVarPrev.FilGain
  Data Store Write : DataStoreWrite  DataStoreName=EcuTMeasFilStVarPrev  DataStoreElements=EcuTMeasFilStVarPrev.FilSt
  Product : Product
  Subtract : Sum  Inputs=+-
  Out1 : Outport
  wires:
  Product/1 -> Add/2
  Subtract/1 -> Product/1
  Input/1 -> Subtract/1
  StateVariable/1 -> Add/1, Subtract/2
  Add/1 -> Data Store Write/1, Out1/1  "EcuTFild"
  Data Store Read/1 -> Product/2

== system ES210A_EcuTMeas/EcuTMeas/EcuTMeasInit/Unauthorized LPF Init SV/Copyright1 ==

== system ES210A_EcuTMeas/EcuTMeas/EcuTMeasPer1/SetNtcSts/Copyright1 ==

== system ES210A_EcuTMeas/EcuTMeas/EcuTMeasPer1/Temperature Range Diagnostic/Copyright1 ==

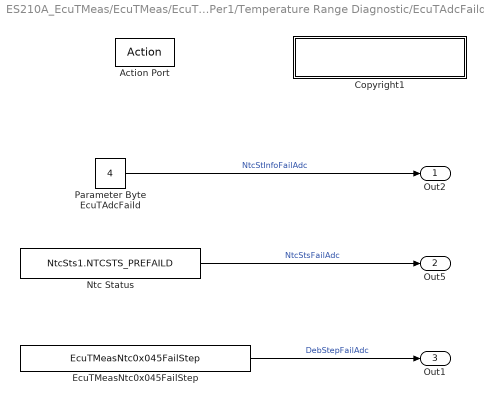
== system ES210A_EcuTMeas/EcuTMeas/EcuTMeasPer1/Temperature Range Diagnostic/EcuTAdcFaild True ==
  Action Port : ActionPort  ActionType=then
  Copyright1 : Subsystem  Description=|  mask(Copyright Information){none=on}
      | Copyright info block.                                               
      |                                                                     
      | Place copyright information at the top of every subsystem in design.
      mask prompts: none "No parameters"
      mask help: Place copyright information at the top of every subsystem in design.
      mask Display:
      | NxtrConf = 'Nexteer Confidential';
      | 
      | sys = bdroot; %handle for the current model ("system")
      | first = get_param(sys,'Created');
      | if(isempty(first))
      |     first = datestr(now,'yyyy');
      | else
      |     first = first(end-3:end);  %year is last four digits
      | end
      | 
      | last = get_param(sys,'LastModifiedDate');
      | if isempty(last)
      |     last = datestr(now,'yyyy');
      | else
      |     last = last(end-3:end);
      | end
      | 
      | if strcmp(first,last)
      |     fprintf('%s\nCopyright  %s Nexteer',NxtrConf,first);
      | else
      |     fprintf('%s\n%s%s-%s Nexteer',NxtrConf,char(169),first,last);
      | end
  EcuTMeasNtc0x045FailStep : Constant  Value=EcuTMeasNtc0x045FailStep
  Ntc Status : Constant  Value=NtcSts1.NTCSTS_PREFAILD  OutDataTypeStr=Enum: NtcSts1
  Parameter Byte EcuTAdcFaild : Constant  Value=4  OutDataTypeStr=uint8
  Out2 : Outport  InitialOutput=2
  Out5 : Outport  Port=2  InitialOutput=NtcSts1.NTCSTS_PREFAILD
  Out1 : Outport  Port=3  InitialOutput=EcuTMeasNtc0x045FailStep
  wires:
  Ntc Status/1 -> Out5/1  "NtcStsFailAdc"
  EcuTMeasNtc0x045FailStep/1 -> Out1/1  "DebStepFailAdc"
  Parameter Byte EcuTAdcFaild/1 -> Out2/1  "NtcStInfoFailAdc"

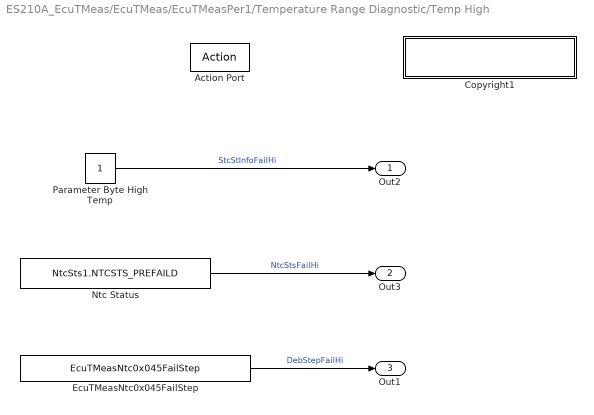
== system ES210A_EcuTMeas/EcuTMeas/EcuTMeasPer1/Temperature Range Diagnostic/Temp High ==
  Action Port : ActionPort  ActionType=elseif
  Copyright1 : Subsystem  Description=|  mask(Copyright Information){none=on}
      | Copyright info block.                                               
      |                                                                     
      | Place copyright information at the top of every subsystem in design.
      mask prompts: none "No parameters"
      mask help: Place copyright information at the top of every subsystem in design.
      mask Display:
      | NxtrConf = 'Nexteer Confidential';
      | 
      | sys = bdroot; %handle for the current model ("system")
      | first = get_param(sys,'Created');
      | if(isempty(first))
      |     first = datestr(now,'yyyy');
      | else
      |     first = first(end-3:end);  %year is last four digits
      | end
      | 
      | last = get_param(sys,'LastModifiedDate');
      | if isempty(last)
      |     last = datestr(now,'yyyy');
      | else
      |     last = last(end-3:end);
      | end
      | 
      | if strcmp(first,last)
      |     fprintf('%s\nCopyright  %s Nexteer',NxtrConf,first);
      | else
      |     fprintf('%s\n%s%s-%s Nexteer',NxtrConf,char(169),first,last);
      | end
  EcuTMeasNtc0x045FailStep : Constant  Value=EcuTMeasNtc0x045FailStep
  Ntc Status : Constant  Value=NtcSts1.NTCSTS_PREFAILD  OutDataTypeStr=Enum: NtcSts1
  Parameter Byte High Temp : Constant  OutDataTypeStr=uint8
  Out2 : Outport  InitialOutput=1
  Out3 : Outport  Port=2  InitialOutput=NtcSts1.NTCSTS_PREFAILD
  Out1 : Outport  Port=3  InitialOutput=EcuTMeasNtc0x045FailStep
  wires:
  Parameter Byte High Temp/1 -> Out2/1  "StcStInfoFailHi"
  EcuTMeasNtc0x045FailStep/1 -> Out1/1  "DebStepFailHi"
  Ntc Status/1 -> Out3/1  "NtcStsFailHi"

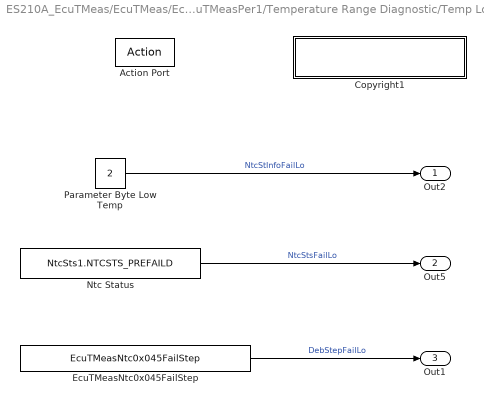
== system ES210A_EcuTMeas/EcuTMeas/EcuTMeasPer1/Temperature Range Diagnostic/Temp Low ==
  Action Port : ActionPort  ActionType=elseif
  Copyright1 : Subsystem  Description=|  mask(Copyright Information){none=on}
      | Copyright info block.                                               
      |                                                                     
      | Place copyright information at the top of every subsystem in design.
      mask prompts: none "No parameters"
      mask help: Place copyright information at the top of every subsystem in design.
      mask Display:
      | NxtrConf = 'Nexteer Confidential';
      | 
      | sys = bdroot; %handle for the current model ("system")
      | first = get_param(sys,'Created');
      | if(isempty(first))
      |     first = datestr(now,'yyyy');
      | else
      |     first = first(end-3:end);  %year is last four digits
      | end
      | 
      | last = get_param(sys,'LastModifiedDate');
      | if isempty(last)
      |     last = datestr(now,'yyyy');
      | else
      |     last = last(end-3:end);
      | end
      | 
      | if strcmp(first,last)
      |     fprintf('%s\nCopyright  %s Nexteer',NxtrConf,first);
      | else
      |     fprintf('%s\n%s%s-%s Nexteer',NxtrConf,char(169),first,last);
      | end
  EcuTMeasNtc0x045FailStep : Constant  Value=EcuTMeasNtc0x045FailStep
  Ntc Status : Constant  Value=NtcSts1.NTCSTS_PREFAILD  OutDataTypeStr=Enum: NtcSts1
  Parameter Byte Low Temp : Constant  Value=2  OutDataTypeStr=uint8
  Out2 : Outport  InitialOutput=2
  Out5 : Outport  Port=2  InitialOutput=NtcSts1.NTCSTS_PREFAILD
  Out1 : Outport  Port=3  InitialOutput=EcuTMeasNtc0x045FailStep
  wires:
  Parameter Byte Low Temp/1 -> Out2/1  "NtcStInfoFailLo"
  EcuTMeasNtc0x045FailStep/1 -> Out1/1  "DebStepFailLo"
  Ntc Status/1 -> Out5/1  "NtcStsFailLo"

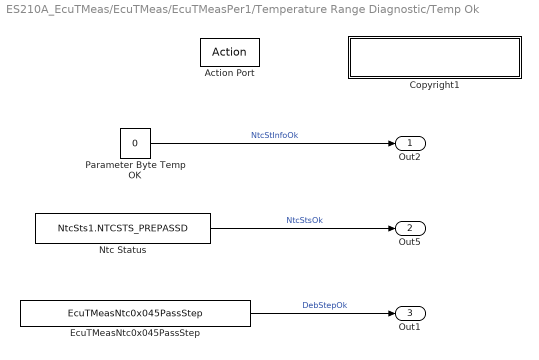
== system ES210A_EcuTMeas/EcuTMeas/EcuTMeasPer1/Temperature Range Diagnostic/Temp Ok ==
  Action Port : ActionPort  ActionType=else
  Copyright1 : Subsystem  Description=|  mask(Copyright Information){none=on}
      | Copyright info block.                                               
      |                                                                     
      | Place copyright information at the top of every subsystem in design.
      mask prompts: none "No parameters"
      mask help: Place copyright information at the top of every subsystem in design.
      mask Display:
      | NxtrConf = 'Nexteer Confidential';
      | 
      | sys = bdroot; %handle for the current model ("system")
      | first = get_param(sys,'Created');
      | if(isempty(first))
      |     first = datestr(now,'yyyy');
      | else
      |     first = first(end-3:end);  %year is last four digits
      | end
      | 
      | last = get_param(sys,'LastModifiedDate');
      | if isempty(last)
      |     last = datestr(now,'yyyy');
      | else
      |     last = last(end-3:end);
      | end
      | 
      | if strcmp(first,last)
      |     fprintf('%s\nCopyright  %s Nexteer',NxtrConf,first);
      | else
      |     fprintf('%s\n%s%s-%s Nexteer',NxtrConf,char(169),first,last);
      | end
  EcuTMeasNtc0x045PassStep : Constant  Value=EcuTMeasNtc0x045PassStep
  Ntc Status : Constant  Value=NtcSts1.NTCSTS_PREPASSD  OutDataTypeStr=Enum: NtcSts1
  Parameter Byte Temp OK : Constant  Value=0  OutDataTypeStr=uint8
  Out2 : Outport  InitialOutput=0
  Out5 : Outport  Port=2  InitialOutput=NtcSts1.NTCSTS_PREPASSD
  Out1 : Outport  Port=3  InitialOutput=EcuTMeasNtc0x045PassStep
  wires:
  Parameter Byte Temp OK/1 -> Out2/1  "NtcStInfoOk"
  EcuTMeasNtc0x045PassStep/1 -> Out1/1  "DebStepOk"
  Ntc Status/1 -> Out5/1  "NtcStsOk"

== system ES210A_EcuTMeas/EcuTMeas/EcuTMeasPer1/Unauthorized LPF/Copyright1 ==

== system ES210A_EcuTMeas/EcuTMeas/EcuTMeasPer1/Temperature Range Diagnostic/EcuTAdcFaild True/Copyright1 ==

== system ES210A_EcuTMeas/EcuTMeas/EcuTMeasPer1/Temperature Range Diagnostic/Temp High/Copyright1 ==

== system ES210A_EcuTMeas/EcuTMeas/EcuTMeasPer1/Temperature Range Diagnostic/Temp Low/Copyright1 ==

== system ES210A_EcuTMeas/EcuTMeas/EcuTMeasPer1/Temperature Range Diagnostic/Temp Ok/Copyright1 ==

== stateflow chart ES210A_EcuTMeas/EcuTMeas/EcuTMeasPer1/SetNtcSts/ISO Fault Debounce Design NOT TO BE IMPLEMENTED IN THIS FDD USED ONLY FOR SIMULATION PURPOSES ==
  note: NTCSTS_PASSD           (0)
      | NTCSTS_FAILD             (1)
      | NTCSTS_PREPASSD   (2)
      | NTCSTS_PREFAILD     (3)
      |
      | SIGQLFR_NORES        (0)
      | SIGQLFR_PASSD         (1)
      | SIGQLFR_FAILD           (2)
  note: Fail step Loop
  note: Pass step Loop
  note: 
  (default) -> (junction 89)
  (junction 89) -> (junction 95) [order 1] : [NtcSts == 3]
  (junction 89) -> (junction 93) [order 2] : [ NtcSts == 2]
  (junction 93) -> (junction 230) [order 2] : {
      | DebCntr = DebCntr - DebStep;
      | }
  (junction 95) -> (junction 216) [order 2] : [DebCntr <= 0]
      | {
      | DebCntr = DebStep;
      | }
  (junction 95) -> (junction 103) [order 1] : [DebCntr > 0]
  (junction 93) -> (junction 123) [order 1] : [(DebCntr - DebStep) <= -32768]
      | {
      | DebCntr = -32768;
      | Qualifier = 1;
      | }
  (junction 230) -> (junction 231)
  (junction 103) -> (junction 216) [order 2] : {
      | DebCntr = DebCntr + DebStep;
      | }
  (junction 216) -> (junction 220) [order 2]
  (junction 216) -> (junction 220) [order 1] : [(DebCntr + DebStep) >=32767]
      | {
      | DebCntr = 32767;
      | Qualifier =2;
      | }
  (junction 103) -> (junction 220) [order 1] : [(DebCntr + DebStep) >=32767]
      | {
      | DebCntr = 32767;
      | Qualifier =2;
      | }
  (junction 220) -> (junction 141)
  (junction 123) -> (junction 141)
  (junction 231) -> (junction 123)
  (junction 141) -> (junction 159)
  data: NtcSts input uint8; Qualifier output uint8 =0; DebStep input uint16; DebCntr output int16
